simulink model "Simulink"  (R2023b)
settings: Solver=FixedStepDiscrete  StartTime=0.0  StopTime=10.0  FixedStep=0.001  RelTol=1e-3
settings Model: Creator=MrLove  LastModifiedBy=MrLove

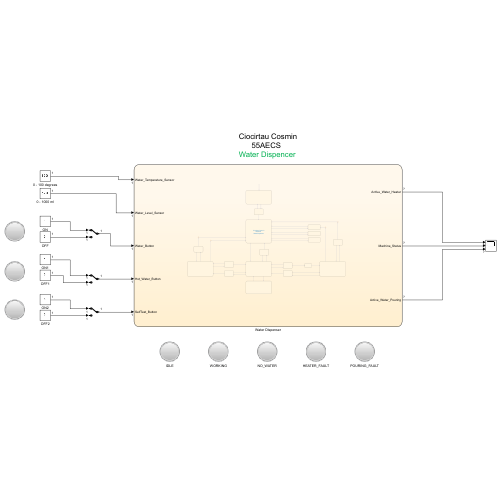
[thumbnail: Simulink's stored preview of the top-level diagram]
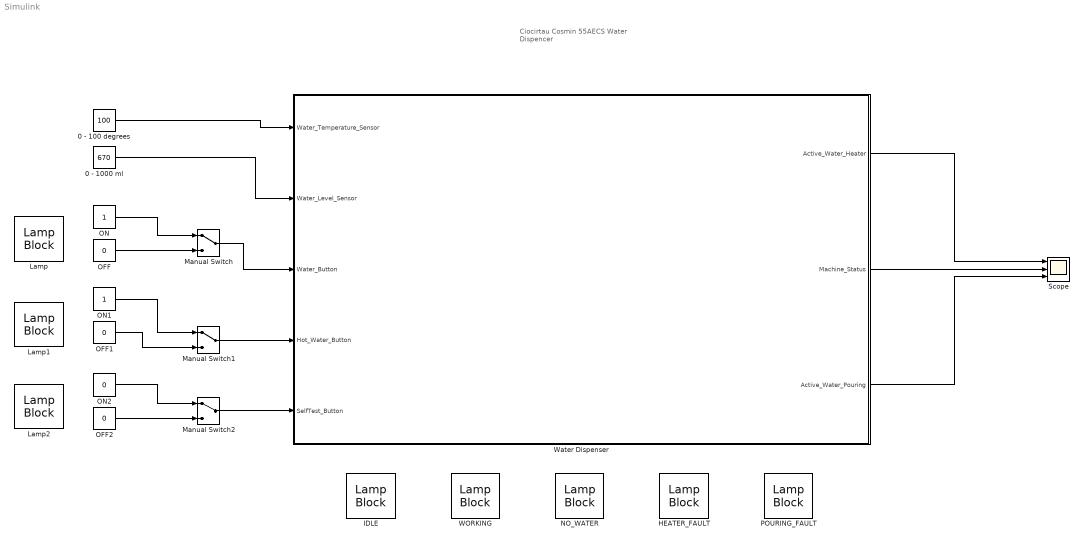
== system Simulink ==
  note: Ciocirtau Cosmin
      | 55AECS
      | Water Dispencer
  0 - 100 degrees : Constant  Value=100
  0 - 1000 ml : Constant  Value=670
  HEATER_FAULT : LampBlock  LabelPosition=Hide
  IDLE : LampBlock  LabelPosition=Hide
  Lamp : LampBlock  LabelPosition=Hide
  Lamp1 : LampBlock  LabelPosition=Hide
  Lamp2 : LampBlock  LabelPosition=Hide
  Manual Switch : ManualSwitch
  Manual Switch1 : ManualSwitch
  Manual Switch2 : ManualSwitch
  NO_WATER : LampBlock  LabelPosition=Hide
  OFF : Constant  Value=0  OutDataTypeStr=boolean
  OFF1 : Constant  Value=0  OutDataTypeStr=boolean
  OFF2 : Constant  Value=0  OutDataTypeStr=boolean
  ON : Constant  OutDataTypeStr=boolean
  ON1 : Constant  OutDataTypeStr=boolean
  ON2 : Constant  Value=0  OutDataTypeStr=boolean
  POURING_FAULT : LampBlock  LabelPosition=Hide
  Scope : Scope  NumInputPorts=3
  WORKING : LampBlock  LabelPosition=Hide
  Water Dispenser : Stateflow chart  TreatAsAtomicUnit=on
  wires:
  Water Dispenser/2(Machine_Status) -> Scope/2
  Water Dispenser/1(Active_Water_Heater) -> Scope/1
  Water Dispenser/3(Active_Water_Pouring) -> Scope/3
  0 - 100 degrees/1 -> Water Dispenser/1(Water_Temperature_Sensor)
  0 - 1000 ml/1 -> Water Dispenser/2(Water_Level_Sensor)
  Manual Switch/1 -> Water Dispenser/3(Water_Button)
  ON/1 -> Manual Switch/1
  OFF/1 -> Manual Switch/2
  ON1/1 -> Manual Switch1/1
  OFF1/1 -> Manual Switch1/2
  Manual Switch1/1 -> Water Dispenser/4(Hot_Water_Button)
  ON2/1 -> Manual Switch2/1
  OFF2/1 -> Manual Switch2/2
  Manual Switch2/1 -> Water Dispenser/5(SelfTest_Button)

== stateflow chart Simulink/Water Dispenser ==
  state REQUIRE_FOR_SELFTEST
  state WAIT_DEBOUCING
  state SELF_TEST
    en:
    SelfTest_Button = 0;
    Active_Water_Pouring = 0;
    note: Ciocirtau Cosmin
        | 55AECS
        | WaterDispenser
  state NO_WATER
    en:
    Machine_Status = 2;
  state POURING_FAULT
    en:
    Machine_Status = 4;
  state HEATER_FAULT
    en:
    Machine_Status = 3;
  state WAIT_DEBOUCING7
  state WAIT_DEBOUCING6
  state WAIT_DEBOUCING5
  state Cold_Water
    en:
    Active_Water_Pouring = 1;
    SelfTest_Button = 0;
    Machine_Status = 1;
  state WAIT_DEBOUCING1
  state WAIT
    en:
    SelfTest_Button = 0;
    Machine_Status = 1;
    Water_Button = 0;
    Hot_Water_Button = 0;
    Active_Water_Heater = 0;
    Active_Water_Pouring = 0;
  state Hot_Water
    en:
    Active_Water_Pouring = 1;
    Active_Water_Heater = 0;
    SelfTest_Button = 0;
    Machine_Status = 1;
  state WAIT_DEBOUCING3
  state Wait_500msec
  state WAIT_DEBOUCING4
  state WAIT_DEBOUCING2
  state IDLE
    en:
    Machine_Status = 0;
    SelfTest_Button = 0;
  note: Sa fac sa mearga doar apa rece,
      | chiar daca nu merge apa calda.
      |
      | Verificarea nivelului de apa mai
      | intai, pentru ca daca nu avem apa,
      | nu mai are rost sa le verificam pe celelalte.
  note: [(Water_Temperature_Sensor >= 99 && after(20, sec)) && (Active_Water_Pouring >= 50 && after(2, sec)) && (Water_Level_Sensor >= 100)]
  (default) -> REQUIRE_FOR_SELFTEST : {SelfTest_Button = 0;
      | Water_Level_Sensor = 0;
      | Water_Temperature_Sensor = 0;
      | SelfTest_Button = 0;
      | Active_Water_Heater = 0;
      | Active_Water_Pouring = 0;
      | Water_Button = 0;
      | Hot_Water_Button = 0;}
  WAIT_DEBOUCING -> REQUIRE_FOR_SELFTEST [order 1] : [SelfTest_Button == 0]
  REQUIRE_FOR_SELFTEST -> WAIT_DEBOUCING : [SelfTest_Button == 1]
  WAIT_DEBOUCING -> SELF_TEST [order 2] : [after(200, msec)]
  (junction 107) -> SELF_TEST
  WAIT_DEBOUCING7 -> (junction 107) [order 1] : [after(200,msec)]
  NO_WATER -> SELF_TEST : [Water_Level_Sensor >= 100]
  (junction 78) -> NO_WATER
  Hot_Water -> (junction 78) [order 1] : [Water_Level_Sensor <= 10]
  SELF_TEST -> NO_WATER [order 1] : [Water_Level_Sensor < 100]
  POURING_FAULT -> SELF_TEST : [Active_Water_Pouring >= 50 && after(2, sec)]
  SELF_TEST -> POURING_FAULT [order 2] : [Active_Water_Pouring <= 50 && after(2, sec)]
  (junction 100) -> SELF_TEST
  WAIT_DEBOUCING6 -> (junction 100) [order 1] : [after(200,msec)]
  HEATER_FAULT -> SELF_TEST : [Water_Temperature_Sensor >= 99 && after(20, sec)]
  (junction 81) -> SELF_TEST
  SELF_TEST -> HEATER_FAULT [order 3] : [Water_Temperature_Sensor < 99 && after(20, sec)]
  Cold_Water -> (junction 81) [order 1] : [Water_Level_Sensor <= 10]
  SELF_TEST -> WAIT [order 4]
  WAIT_DEBOUCING5 -> SELF_TEST [order 2] : [after(200,msec)]
  WAIT_DEBOUCING7 -> Hot_Water [order 2] : [SelfTest_Button == 0]
  Hot_Water -> WAIT_DEBOUCING7 [order 2] : [SelfTest_Button == 1]
  WAIT_DEBOUCING6 -> Cold_Water [order 2] : [SelfTest_Button == 0]
  Cold_Water -> WAIT_DEBOUCING6 [order 2] : [SelfTest_Button == 1]
  WAIT_DEBOUCING5 -> WAIT [order 1] : [SelfTest_Button == 0]
  WAIT -> WAIT_DEBOUCING5 [order 4] : [SelfTest_Button == 1]
  WAIT_DEBOUCING1 -> Cold_Water [order 2] : [Water_Button == 1]
  WAIT_DEBOUCING3 -> WAIT [order 1] : [Hot_Water_Button == 0]
  WAIT_DEBOUCING1 -> WAIT [order 1] : [after(200, msec)]
  Wait_500msec -> Hot_Water : [after(500, msec)]
  WAIT_DEBOUCING3 -> Wait_500msec [order 2] : [after(200, msec)]
      | {Active_Water_Heater = 1;}
  Cold_Water -> WAIT_DEBOUCING1 [order 3] : [Water_Button == 0]
  WAIT -> WAIT_DEBOUCING3 [order 3] : [Hot_Water_Button == 1]
  WAIT_DEBOUCING4 -> Hot_Water [order 1] : [Hot_Water_Button == 1]
  WAIT_DEBOUCING2 -> WAIT [order 2] : [Water_Button == 0]
  WAIT_DEBOUCING4 -> WAIT [order 2] : [after(200, msec)]
  WAIT_DEBOUCING2 -> Cold_Water [order 1] : [after(200, msec)]
  WAIT -> WAIT_DEBOUCING2 [order 1] : [Water_Button == 1]
  Hot_Water -> WAIT_DEBOUCING4 [order 3] : [Hot_Water_Button == 0]
  IDLE -> WAIT : [Hot_Water_Button == 1 || Water_Button == 1 || SelfTest_Button == 1]
  WAIT -> IDLE [order 2] : [after(120, sec)]
  data: Active_Water_Heater output; Machine_Status output; Water_Temperature_Sensor input; Water_Level_Sensor input; Active_Water_Pouring output; Water_Button input; Hot_Water_Button input; SelfTest_Button input
